simulink model "piddcs"  (R2023b)
settings: Solver=VariableStepAuto  StartTime=0.0  StopTime=10.0  RelTol=1e-3
settings Model: Creator=LEGION  LastModifiedBy=LEGION

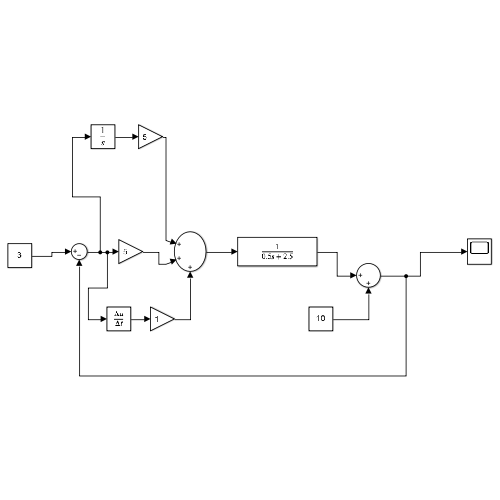
[thumbnail: Simulink's stored preview of the top-level diagram]
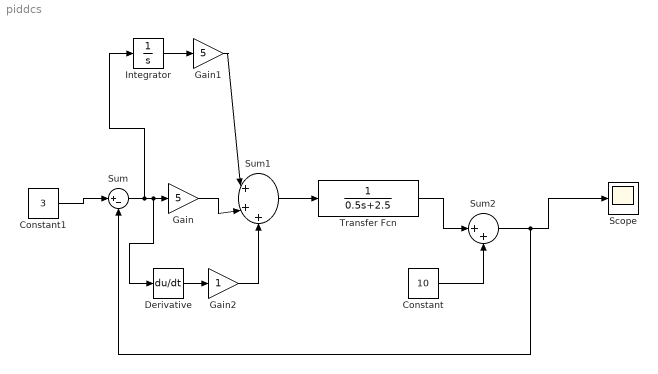
== system piddcs ==
  Constant : Constant  Value=10
  Constant1 : Constant  Value=3
  Derivative : Derivative
  Gain : Gain  Gain=5
  Gain1 : Gain  Gain=5
  Gain2 : Gain
  Integrator : Integrator
  Scope : Scope
  Sum : Sum  Inputs=|+-
  Sum1 : Sum  Inputs=|+++
  Sum2 : Sum  Inputs=|++
  Transfer Fcn : TransferFcn  Denominator=[0.5 2.5]
  wires:
  Constant1/1 -> Sum/1
  Sum/1 -> Integrator/1, Derivative/1, Gain/1
  Gain/1 -> Sum1/2
  Sum1/1 -> Transfer Fcn/1
  Gain1/1 -> Sum1/1
  Integrator/1 -> Gain1/1
  Derivative/1 -> Gain2/1
  Gain2/1 -> Sum1/3
  Constant/1 -> Sum2/2
  Transfer Fcn/1 -> Sum2/1
  Sum2/1 -> Sum/2, Scope/1
